simulink model "ModelHalfCarDOF5"  (R2022b)
settings: Solver=ode4  StartTime=0.0  StopTime=100.0  FixedStep=10^-3  RelTol=1e-3
values from neighbouring files (symbols this model uses):
  cs1 = 991    [OptimizedParamDOF5.m]
  cs2 = 996    [OptimizedParamDOF5.m]
  css = 3344    [ModelFixedParamDOF5.m]
  Is = 130    [ModelFixedParamDOF5.m]
  kp1 = 175500    [ModelFixedParamDOF5.m]
  kp2 = 175500    [ModelFixedParamDOF5.m]
  ks1 = 18222    [OptimizedParamDOF5.m]
  ks2 = 19516    [OptimizedParamDOF5.m]
  kss = 68794    [ModelFixedParamDOF5.m]
  l1 = 1.011    [ModelFixedParamDOF5.m]
  l2 = 1.803    [ModelFixedParamDOF5.m]
  m1 = 417    [ModelFixedParamDOF4.m]    (also in ModelFixedParamDOF5.m = 40)
  m2 = 15    [ModelFixedParamDOF4.m]    (also in ModelFixedParamDOF5.m = 35.5)
  mc = 441    [ModelFixedParamDOF3.m]    (also in ModelFixedParamDOF5.m = 75)
  ms = 237    [ModelFixedParamDOF2.m]    (also in ModelFixedParamDOF3.m = 35; ModelFixedParamDOF5.m = 730)
  r = 0.25    [ModelFixedParamDOF5.m]
  road_front_wheel = M.'    [LoadRoadScript.m]
settings Model: Creator=ALINA  LastModifiedBy=andre
settings SolverCC: AlgebraicLoopSolver=TrustRegion
settings DataIOCC: ReturnWorkspaceOutputs=off
settings OptimizationCC: LifeSpan=inf
settings DebuggingCC: UnconnectedInputMsg=warning  UnconnectedOutputMsg=warning  UnconnectedLineMsg=warning  SFUnexpectedBacktrackingDiag=warning  SFNoUnconditionalDefaultTransitionDiag=warning  SFMachineParentedDataDiag=warning  ArithmeticOperatorsInVariantConditions=warning
settings ModelReferenceCC: EnableRefExpFcnMdlSchedulingChecks=on
settings SFSimCC: SimUseLocalCustomCode=off  CustomCodeUndefinedFunction=UseInterfaceOnly
settings RTWCC: RTWUseLocalCustomCode=off  DLArmComputeVersion=19.05
settings CodeAppCC: StateflowObjectComments=on
settings GRTTargetCC: TargetLangStandard=C89/C90 (ANSI)
settings ConfigComp: CovMetricSettings=dw  CovSaveCumulativeToWorkspaceVar=on  CovSaveSingleToWorkspaceVar=on  CovExternalEMLEnable=off

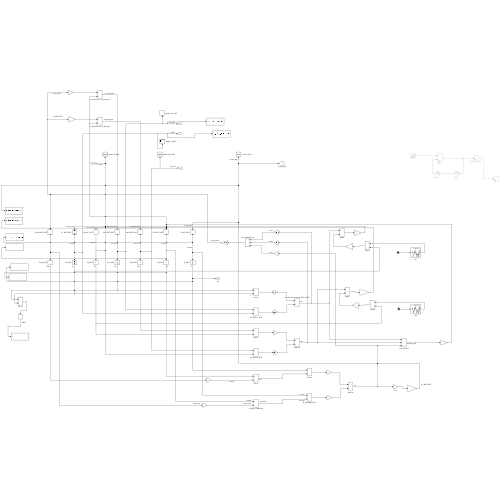
[thumbnail: Simulink's stored preview of the top-level diagram]
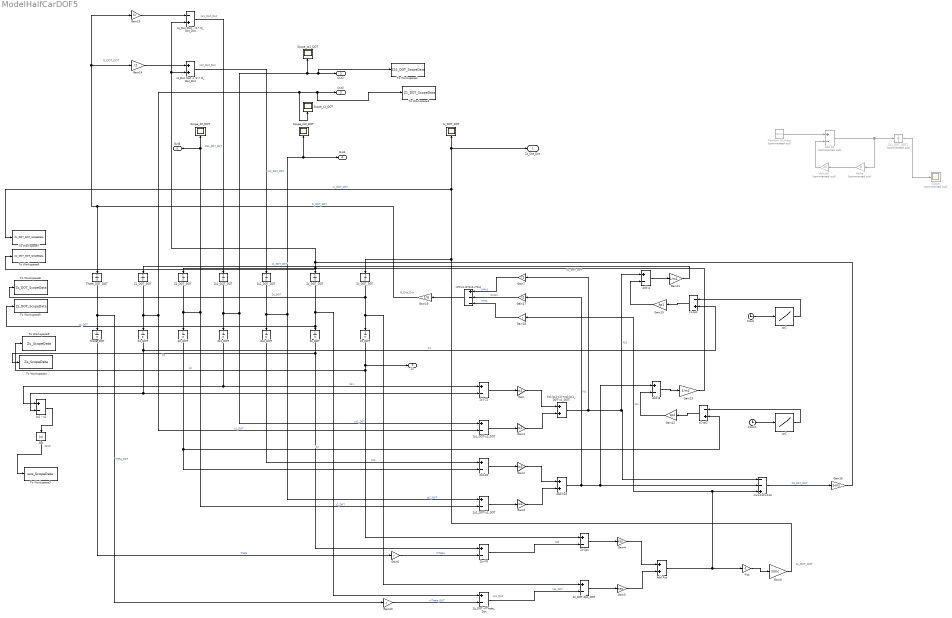
== system ModelHalfCarDOF5 ==
  note: SWS
  note: zps_Dot
  note: O_DOT_DOT
  note: zs2_Dot_Dot
  note: zs1_Dot_Dot
  note: O_Dot_Dot
  note: Zc_DOT_DOT
  -Fs1-Fs2+Fs3 : Sum  Inputs=--+
  -Fss : Gain  Gain=-1
  Abs : Abs  SaturateOnIntegerOverflow=off
  Add A : Sum  Inputs=+-
  Add A1 : Sum  Commented=on  Inputs=+-
  Add B : Sum  Inputs=+-
  Add Fs2 : Sum
  Add Fss : Sum
  Alpha : Gain  Commented=on  Gain=8
  Clock : Clock
  Clock1 : Clock
  Gain : Gain  Gain=ks1
  Gain1 : Gain  Gain=cs1
  Gain10 : Gain  Gain=kp1
  Gain11 : Gain  Gain=1/m1
  Gain12 : Gain  Gain=kp2
  Gain13 : Gain  Gain=1/m2
  Gain14 : Gain  Gain=l2
  Gain15 : Gain  Gain=l1
  Gain16 : Gain  Gain=1/ms
  Gain17 : Gain  Gain=l2
  Gain18 : Gain  Gain=r
  Gain19 : Gain  Gain=1/Is
  Gain2 : Gain  Gain=ks2
  Gain20 : Gain  Gain=r
  Gain3 : Gain  Gain=cs2
  Gain4 : Gain  Gain=kss
  Gain5 : Gain  Gain=css
  Gain6 : Gain  Gain=r
  Gain7 : Gain  Gain=l1
  Gain9 : Gain  Gain=1/mc
  Random Number : RandomNumber  Commented=on  SampleTime=0.1
  Scope : Scope  Commented=on
  Scope_Z2_DOT : Scope
  Scope_z1_DOT : Scope
  Scope_zs1_DOT : Scope
  Scope_zs2_DOT : Scope
  Theta_DOT : Integrator
  Theta_DOT_DOT : Integrator
  To Workspace1 : ToWorkspace  VariableName=Z1_DOT_ScopeData  SaveFormat=Structure With Time  SampleTime=-1
  To Workspace2 : ToWorkspace  VariableName=ZS1_DOT_ScopeData  SaveFormat=Structure With Time  SampleTime=-1
  To Workspace3 : ToWorkspace  VariableName=sws_ScopeData  SaveFormat=Structure With Time  SampleTime=-1
  To Workspace4 : ToWorkspace  VariableName=Zs_ScopeData  SaveFormat=Structure With Time  SampleTime=-1
  To Workspace5 : ToWorkspace  VariableName=Zs_DOT_ScopeData  SaveFormat=Structure With Time  SampleTime=-1
  To Workspace6 : ToWorkspace  VariableName=Zs_DOT_DOT_ScopeData  SaveFormat=Structure With Time  SampleTime=-1
  To Workspace7 : ToWorkspace  VariableName=Zc_DOT_DOT_ScopeData  SaveFormat=Structure With Time  SampleTime=-1
  To Workspace8 : ToWorkspace  VariableName=Zc_DOT_ScopeData  SaveFormat=Structure With Time  SampleTime=-1
  To Workspace9 : ToWorkspace  VariableName=Zc_ScopeData  SaveFormat=Structure With Time  SampleTime=-1
  Velocity : Gain  Commented=on  Gain=20
  Z1_DOT : Integrator
  Z1_DOT_DOT : Integrator
  Z2_DOT : Integrator
  Z2_DOT_DOT : Integrator
  Zc-Zps : Sum  Inputs=+-
  Zc_DOT : Integrator
  Zc_DOT-Zps_DOT : Sum  Inputs=+-
  Zc_DOT_DOT : Integrator
  Zs-r*O : Sum  Inputs=+-
  Zs1-Z1 : Sum  Inputs=+-
  Zs1_DOT : Integrator
  Zs1_DOT-z1_DOT : Sum  Inputs=+-
  Zs1_DOT_DOT : Integrator
  Zs2-Z2 : Sum  Inputs=+-
  Zs2_DOT : Integrator
  Zs2_DOT-z2_DOT : Sum  Inputs=+-
  Zs2_DOT_DOT : Integrator
  Zs2_DOT_DOT1 : Integrator  Commented=on
  Zs_DOT : Integrator
  Zs_DOT-r*Theta_Dot : Sum  Inputs=+-
  Zs_DOT_DOT : Integrator
  ks1(zs1-z1)+cs1(zs1_DOT-z1_DOT) : Sum
  l1*Fs1-l2*Fs2-r*Fss : Sum  Inputs=+--
  z1-zp1 : Sum  Inputs=-+
  z2-zp2 : Sum  Inputs=-+
  zc_DOT_DOT : Scope
  zp1 : Lookup_n-D  NumberOfTableDimensions=1  LookupTableObject=road_front_wheel  BreakpointsForDimension1=[1:100]  Table=road_front_wheel  InternalRulePriority=Speed  RndMeth=Simplest
  zp2 : Lookup_n-D  NumberOfTableDimensions=1  LookupTableObject=road_front_wheel  BreakpointsForDimension1=[1:100]  Table=road_front_wheel  InternalRulePriority=Speed  RndMeth=Simplest
  zs1 - z1 : Sum  Inputs=+-
  zs_Dot_Dot + l2 * O_Dot_Dot : Sum
  zs_Dot_Dot - l1 * O_Dot_Dot : Sum  Inputs=-+
  Zc_Dot_Dot : Outport
  Out2 : Outport  Port=2
  Out3 : Outport  Port=3
  Out4 : Outport  Port=4
  Out5 : Outport  Port=5
  Zc : Outport  Port=6
  wires:
  Z1_DOT_DOT/1 -> Scope_z1_DOT/1, To Workspace1/1, Out3/1, Zs1_DOT-z1_DOT/2, Z1_DOT/1  "z1_DOT"
  Z2_DOT_DOT/1 -> Z2_DOT/1, Zs2_DOT-z2_DOT/2, Out5/1, Scope_Z2_DOT/1  "z2_DOT"
  Zs1_DOT_DOT/1 -> Zs1_DOT/1, Scope_zs1_DOT/1, To Workspace2/1, Out2/1, Zs1_DOT-z1_DOT/1  "zs1_DOT"
  Zs2_DOT_DOT/1 -> Zs2_DOT/1, Out4/1, Scope_zs2_DOT/1, Zs2_DOT-z2_DOT/1  "zs2_DOT"
  Zs_DOT_DOT/1 -> Zs_DOT-r*Theta_Dot/1, To Workspace5/1, Zs_DOT/1  "zs_DOT"
  Zc_DOT_DOT/1 -> Zc_DOT/1, Zc_DOT-Zps_DOT/1, To Workspace8/1  "Zc_DOT"
  Zs1_DOT/1 -> zs1 - z1/1, Zs1-Z1/1  "Zs1"
  Z1_DOT/1 -> Zs1-Z1/2, zs1 - z1/2, z1-zp1/2  "Z1"
  Zs1-Z1/1 -> Gain/1
  Gain/1 -> ks1(zs1-z1)+cs1(zs1_DOT-z1_DOT)/1
  Zs1_DOT-z1_DOT/1 -> Gain1/1
  Gain1/1 -> ks1(zs1-z1)+cs1(zs1_DOT-z1_DOT)/2
  ks1(zs1-z1)+cs1(zs1_DOT-z1_DOT)/1 -> Gain7/1, Add A/1, -Fs1-Fs2+Fs3/1  "Fs1"
  Zs2-Z2/1 -> Gain2/1
  Gain2/1 -> Add Fs2/1
  Zs2_DOT-z2_DOT/1 -> Gain3/1
  Gain3/1 -> Add Fs2/2
  Add Fs2/1 -> Add B/1, -Fs1-Fs2+Fs3/2, Gain17/1  "Fs2"
  Zs2_DOT/1 -> Zs2-Z2/1  "Zs2"
  Z2_DOT/1 -> Zs2-Z2/2, z2-zp2/2  "Z2"
  Zc-Zps/1 -> Gain4/1
  Gain4/1 -> Add Fss/1
  Zc_DOT-Zps_DOT/1 -> Gain5/1
  Gain5/1 -> Add Fss/2
  Zs-r*O/1 -> Zc-Zps/2  "Zps"
  Zs_DOT/1 -> Zs-r*O/1, To Workspace4/1  "Zs"
  Zc_DOT/1 -> Zc/1, To Workspace9/1, Zc-Zps/1  "Zc"
  Zs_DOT-r*Theta_Dot/1 -> Zc_DOT-Zps_DOT/2  "zps_DOT"
  Add Fss/1 -> -Fs1-Fs2+Fs3/3, Gain18/1, -Fss/1  "Fss"
  -Fs1-Fs2+Fs3/1 -> Gain16/1  "ZS_DOT_DOT"
  -Fss/1 -> Gain9/1
  Gain9/1 -> Zc_DOT_DOT/1, To Workspace7/1, Zc_Dot_Dot/1, zc_DOT_DOT/1  "zc_DOT_DOT"
  Gain10/1 -> Add A/2
  z1-zp1/1 -> Gain10/1
  Add A/1 -> Gain11/1
  Gain11/1 -> Z1_DOT_DOT/1  "z1_DOT_DOT"
  Gain12/1 -> Add B/2
  z2-zp2/1 -> Gain12/1
  Add B/1 -> Gain13/1
  Gain13/1 -> Z2_DOT_DOT/1  "Z2_DOT_DOT"
  Gain15/1 -> zs_Dot_Dot - l1 * O_Dot_Dot/1
  zs_Dot_Dot - l1 * O_Dot_Dot/1 -> Zs1_DOT_DOT/1  "ZS1_DOT_DOT"
  Gain14/1 -> zs_Dot_Dot + l2 * O_Dot_Dot/1
  zs_Dot_Dot + l2 * O_Dot_Dot/1 -> Zs2_DOT_DOT/1  "zs2_DOT_DOT"
  Random Number/1 -> Add A1/1
  Add A1/1 -> Alpha/1, Zs2_DOT_DOT1/1
  Zs2_DOT_DOT1/1 -> Scope/1
  Alpha/1 -> Velocity/1
  Velocity/1 -> Add A1/2
  zp2/1 -> z2-zp2/1
  zp1/1 -> z1-zp1/1
  Gain16/1 -> zs_Dot_Dot + l2 * O_Dot_Dot/2, zs_Dot_Dot - l1 * O_Dot_Dot/2, To Workspace6/1, Zs_DOT_DOT/1
  Theta_DOT_DOT/1 -> Gain20/1, Theta_DOT/1  "Theta_DOT"
  Theta_DOT/1 -> Gain6/1  "Theta"
  Gain6/1 -> Zs-r*O/2  "r*Theta"
  Gain19/1 -> Theta_DOT_DOT/1, Gain15/1, Gain14/1  "O_DOT_DOT"
  Gain7/1 -> l1*Fs1-l2*Fs2-r*Fss/1  "l1*Fs1"
  Gain17/1 -> l1*Fs1-l2*Fs2-r*Fss/2  "l2*Fs2"
  Gain18/1 -> l1*Fs1-l2*Fs2-r*Fss/3  "r*Fss"
  l1*Fs1-l2*Fs2-r*Fss/1 -> Gain19/1
  Gain20/1 -> Zs_DOT-r*Theta_Dot/2  "r*Theta_DOT"
  Clock/1 -> zp1/1
  Clock1/1 -> zp2/1
  zs1 - z1/1 -> Abs/1
  Abs/1 -> To Workspace3/1
